simulink model "simulation"  (R2015b)
settings: Solver=VariableStepAuto  StartTime=0.0  StopTime=10  RelTol=1e-3
values from neighbouring files (symbols this model uses):
  bBall = block.DialogPrm(2).Data    [VirtualEnvironment0.m]    (also in VirtualEnvironment1.m; VirtualEnvironment2.m; VirtualEnvironment3.m; VirtualEnvironment4.m)
  bWall = block.DialogPrm(2).Data    [HapticController.m]    (also in Initiation.m = 0; VirtualEnvironment5.m)
  dimensions = block.DialogPrm(5).Data    [HapticController.m]    (also in VirtualObject.m = block.DialogPrm(3).Data)
  inertia = block.DialogPrm(2).Data    [VirtualObject.m]
  kWall = block.DialogPrm(1).Data    [HapticController.m]    (also in Initiation.m = 5000; VirtualEnvironment5.m)
  mass = block.DialogPrm(1).Data    [VirtualObject.m]
  nWall = block.DialogPrm(6).Data    [Controller1.m]    (also in HapticController.m = block.DialogPrm(3).Data; Initial_Conditions.m = -1; Initiation.m = -1; MoreConservative.m = block.DialogPrm(5).Data)
  pBall0 = block.DialogPrm(7).Data    [HapticController.m]
  pose0 = block.DialogPrm(2).Data    [Controller_more.m]    (also in VirtualObject.m = block.DialogPrm(5).Data)
  pose_dot0 = block.DialogPrm(6).Data    [VirtualObject.m]
  pWall = block.DialogPrm(5).Data    [Controller1.m]    (also in HapticController.m = block.DialogPrm(4).Data; Parameters.m = 0; VirtualEnvironment.m = block.DialogPrm(4).Data)
  tsampling = block.DialogPrm(3).Data    [Controller.m]    (also in Controller1.m; Controller_more.m = block.DialogPrm(4).Data; HapticController.m = block.DialogPrm(6).Data; Initial_Conditions.m = 0.001)
  vBall0 = block.DialogPrm(8).Data    [HapticController.m]
undefined symbols (not defined in the file or in its folder): mBall
libraries: simulink x2
settings Model: Creator=TOSHIBA  LastModifiedBy=TOSHIBA

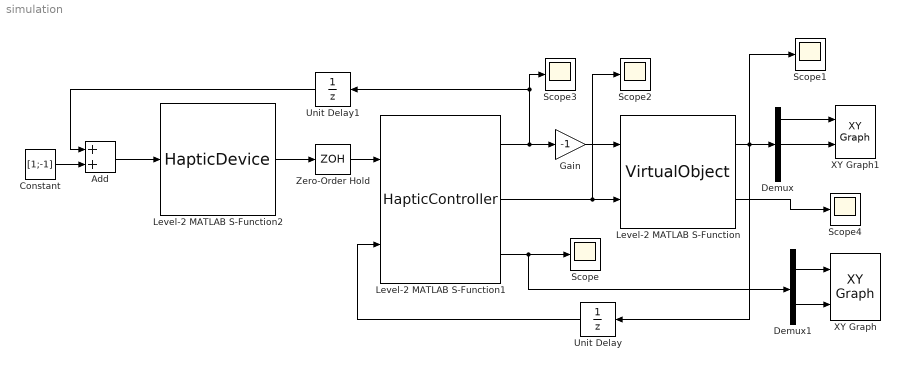
== system simulation ==
  Add : Sum
  Constant : Constant  Value=[1;-1]
  Demux : Demux  Outputs=3
  Demux1 : Demux  Outputs=2
  Gain : Gain  Gain=-1
  Level-2 MATLAB S-Function : M-S-Function  FunctionName=VirtualObject  Parameters=mass,inertia,dimensions,tsampling,pose0,pose_dot0
  Level-2 MATLAB S-Function1 : M-S-Function  FunctionName=HapticController  Parameters=kWall,bWall,nWall,pWall,dimensions,tsampling,pBall0,vBall0
  Level-2 MATLAB S-Function2 : M-S-Function  FunctionName=HapticDevice  Parameters=mBall,bBall,vBall0,dimensions
  Scope{,1..4} (5 alike) : Scope
  Unit Delay : UnitDelay  InitialCondition=pose0  SampleTime=tsampling
  Unit Delay1 : UnitDelay  InitialCondition=[0;0]  SampleTime=tsampling
  XY Graph : simulink/Sinks/XY Graph  xmin=0  xmax=5.5  ymin=0  ymax=5.5  st=tsampling
  XY Graph1 : simulink/Sinks/XY Graph  xmin=2  xmax=4  ymin=-1  ymax=0  st=tsampling
  Zero-Order Hold : ZeroOrderHold  SampleTime=tsampling
  wires:
  Level-2 MATLAB S-Function/1 -> Scope1/1, Unit Delay/1, Demux/1
  Level-2 MATLAB S-Function2/1 -> Zero-Order Hold/1
  Unit Delay/1 -> Level-2 MATLAB S-Function1/2
  Level-2 MATLAB S-Function1/3 -> Demux1/1, Scope/1
  Constant/1 -> Add/2
  Add/1 -> Level-2 MATLAB S-Function2/1
  Zero-Order Hold/1 -> Level-2 MATLAB S-Function1/1
  Demux1/1 -> XY Graph/1
  Demux1/2 -> XY Graph/2
  Demux/2 -> XY Graph1/2
  Demux/1 -> XY Graph1/1
  Level-2 MATLAB S-Function1/1 -> Scope3/1, Unit Delay1/1, Gain/1
  Unit Delay1/1 -> Add/1
  Level-2 MATLAB S-Function1/2 -> Scope2/1, Level-2 MATLAB S-Function/2
  Gain/1 -> Level-2 MATLAB S-Function/1
  Level-2 MATLAB S-Function/2 -> Scope4/1
